simulink model "sharedControlBackup"  (R2018a)
settings: Solver=FixedStepAuto  StartTime=0.0  StopTime=200  FixedStep=.1  RelTol=1e-3
values from neighbouring files (symbols this model uses):
  a = -real(s1) + imag(s1)/tan(angle(s1+b) - theta)    [RLDesignJoystick.m]    (also in gainPlot.m = 10)
  a1 = b1/K    [RLDesignJoystick.m]
  b = 1.2*bb/I    (= 0.4)    [RLDesignJoystick.m]    (also in gainPlot.m)
  b1 = -real(s1)/150    [RLDesignJoystick.m]
  K0 = abs(s1+a)/abs(Gs1)/abs(s1+b)    [RLDesignJoystick.m]    (also in gainPlot.m = 0.5)
  K1 = 1/abs(Gs1)    [RLDesignJoystick.m]
undefined symbols (not defined in the file or in its folder): a2, b2, K2, U
libraries: robotlib x4, simulink x1
settings Model: Creator=transmogrifierlight  LastModifiedBy=transmogrifier

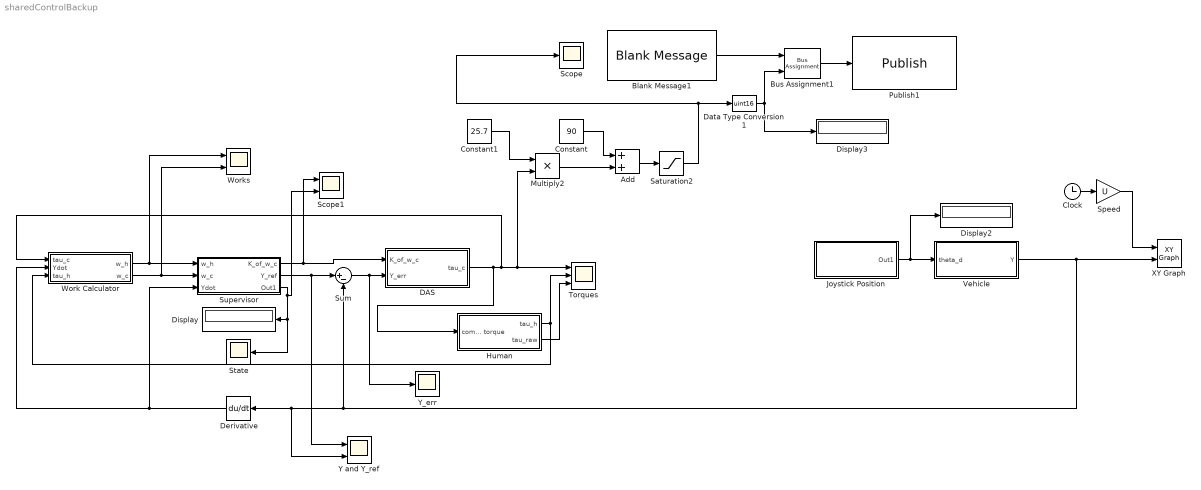
== system sharedControlBackup ==
  Add : Sum
  Blank Message1 : robotlib/Blank Message  SourceLibraryInfo=This block requires Robotics System Toolbox  messageType=std_msgs/UInt16  SampleTime=inf
      settings: SourceProductBaseCode=RO
  Bus Assignment1 : BusAssignment  AssignedSignals=Data
  Clock : Clock
  Constant : Constant  Value=90
  Constant1 : Constant  Value=25.7
  DAS : Subsystem
  Data Type Conversion1 : DataTypeConversion  OutDataTypeStr=uint16
  Derivative : Derivative
  Display : Display
  Display2 : Display
  Display3 : Display
  Human : Subsystem
  Joystick Position : Subsystem
  Multiply2 : Product
  Publish1 : robotlib/Publish  SourceLibraryInfo=This block requires Robotics System Toolbox  topicSource=Select from ROS network  topic=/yMotor  messageType=std_msgs/UInt16  messageQueueLength=1
      settings: SourceProductBaseCode=RO
  Saturation2 : Saturate  UpperLimit=140  LowerLimit=40
  Scope : Scope
  Scope1 : Scope  NumInputPorts=2
  Speed : Gain  Gain=U
  State : Scope
  Sum : Sum  Inputs=|+-
  Supervisor : Subsystem  mask{gamma_1_sq=0.2, gamma_2_sq=0.1, a_d=10, b_d=0.4, sigma_sq=0.1, delta_y=4, K3=0.5}
      mask prompts: gamma_1_sq "DAS Threshold"; gamma_2_sq "Human Threshold"; a_d "a"; b_d "b"; sigma_sq "Lane Change Threshold"; delta_y "Lane Change Delta"; K3 "K0"
  Torques : Scope  NumInputPorts=3
  Vehicle : Subsystem
  Work Calculator : Subsystem  mask{DT=4}
      mask prompts: DT "Time Window"
  Works : Scope  NumInputPorts=2
  XY Graph : simulink/Sinks/XY Graph  xmin=-10  xmax=U*200  ymin=-10  ymax=10  st=-1
  Y and Y_ref : Scope  NumInputPorts=2
  Y_err : Scope
  wires:
  Work Calculator/1(w_h) -> Works/1, Supervisor/1(w_h)
  Work Calculator/2(w_c) -> Works/2, Supervisor/2(w_c)
  Supervisor/1(K_of_w_c) -> Scope1/1, DAS/1("K_of_w_c ")
  Supervisor/2(Y_ref) -> Y and Y_ref/1, Sum/1
  Sum/1 -> Y_err/1, DAS/2(Y_err)
  Clock/1 -> Speed/1
  Speed/1 -> XY Graph/1
  Vehicle/1(Y) -> Sum/2, Y and Y_ref/2, Derivative/1, XY Graph/2
  Derivative/1 -> Work Calculator/2(Ydot), Supervisor/3(Ydot)
  Supervisor/3(Out1) -> Scope1/2, State/1, Display/1
  Human/1(tau_h) -> Work Calculator/3(tau_h), Torques/2
  Joystick Position/1(Out1) -> Vehicle/1(theta_d), Display2/1
  Bus Assignment1/1 -> Publish1/1
  Blank Message1/1 -> Bus Assignment1/1
  Data Type Conversion1/1 -> Bus Assignment1/2, Display3/1
  Constant1/1 -> Multiply2/1
  DAS/1(tau_c) -> Human/1(command torque), Work Calculator/1(tau_c), Multiply2/2, Torques/1
  Multiply2/1 -> Add/2
  Add/1 -> Saturation2/1
  Constant/1 -> Add/1
  Saturation2/1 -> Scope/1, Data Type Conversion1/1
  Human/2(tau_raw) -> Torques/3

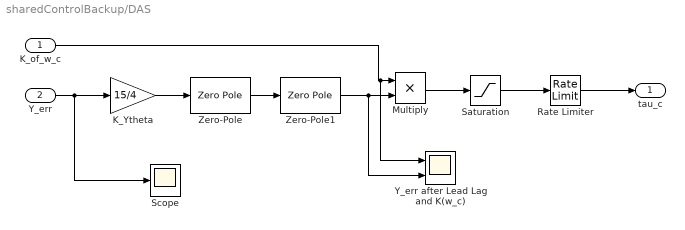
== system sharedControlBackup/DAS ==
  "K_of_w_c " : Inport
  Y_err : Inport  Port=2
  K_Ytheta : Gain  Gain=15/4
  Multiply : Product
  Rate Limiter : RateLimiter  RisingSlewLimit=3  FallingSlewLimit=-3  SampleTimeMode=inherited
  Saturation : Saturate  UpperLimit=5  LowerLimit=-5
  Scope : Scope
  Y_err after Lead Lag and K(w_c) : Scope  NumInputPorts=2
  Zero-Pole : ZeroPole  Zeros=[-b]  Poles=[-a]  Gain=[K0]
  Zero-Pole1 : ZeroPole  Zeros=[-b1]  Poles=[-a1]  Gain=[K1]
  tau_c : Outport
  wires:
  Y_err/1 -> Scope/1, K_Ytheta/1
  Saturation/1 -> Rate Limiter/1
  Multiply/1 -> Saturation/1
  "K_of_w_c "/1 -> Y_err after Lead Lag and K(w_c)/1, Multiply/1
  Zero-Pole/1 -> Zero-Pole1/1
  K_Ytheta/1 -> Zero-Pole/1
  Zero-Pole1/1 -> Y_err after Lead Lag and K(w_c)/2, Multiply/2
  Rate Limiter/1 -> tau_c/1

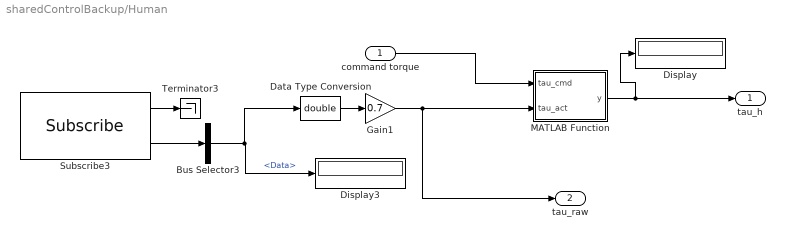
== system sharedControlBackup/Human ==
  command torque : Inport
  Bus Selector3 : BusSelector  OutputSignals=Data
  Data Type Conversion : DataTypeConversion  OutDataTypeStr=double
  Display : Display
  Display3 : Display
  Gain1 : Gain  Gain=0.7
  MATLAB Function : MATLAB Function  TreatAsAtomicUnit=on
  Subscribe3 : robotlib/Subscribe  SourceLibraryInfo=This block requires Robotics System Toolbox  topicSource=Select from ROS network  topic=/yCurrent  messageType=std_msgs/Float32  sampleTime=-1  messageQueueLength=1
      settings: SourceProductBaseCode=RO
  Terminator3 : Terminator
  tau_h : Outport
  tau_raw : Outport  Port=2
  wires:
  Subscribe3/1 -> Terminator3/1
  Data Type Conversion/1 -> Gain1/1
  Subscribe3/2 -> Bus Selector3/1
  Bus Selector3/1 -> Data Type Conversion/1, Display3/1  "<Data>"
  Gain1/1 -> tau_raw/1, MATLAB Function/2(tau_act)
  command torque/1 -> MATLAB Function/1(tau_cmd)
  MATLAB Function/1(y) -> Display/1, tau_h/1

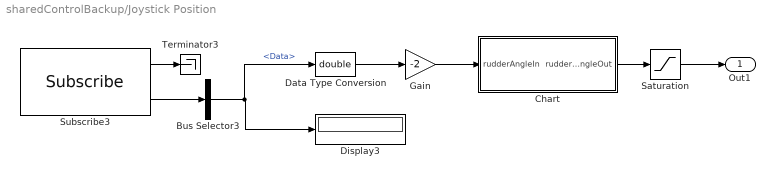
== system sharedControlBackup/Joystick Position ==
  Bus Selector3 : BusSelector  OutputSignals=Data
  Chart : Stateflow chart  TreatAsAtomicUnit=on
  Data Type Conversion : DataTypeConversion  OutDataTypeStr=double
  Display3 : Display
  Gain : Gain  Gain=-2
  Saturation : Saturate  UpperLimit=20  LowerLimit=-20
  Subscribe3 : robotlib/Subscribe  SourceLibraryInfo=This block requires Robotics System Toolbox  topicSource=Select from ROS network  topic=/yPos  messageType=std_msgs/Float32  sampleTime=-1  messageQueueLength=1
      settings: SourceProductBaseCode=RO
  Terminator3 : Terminator
  Out1 : Outport
  wires:
  Subscribe3/2 -> Bus Selector3/1
  Subscribe3/1 -> Terminator3/1
  Bus Selector3/1 -> Data Type Conversion/1, Display3/1  "<Data>"
  Data Type Conversion/1 -> Gain/1
  Gain/1 -> Chart/1(rudderAngleIn)
  Chart/1(rudderAngleOut) -> Saturation/1
  Saturation/1 -> Out1/1

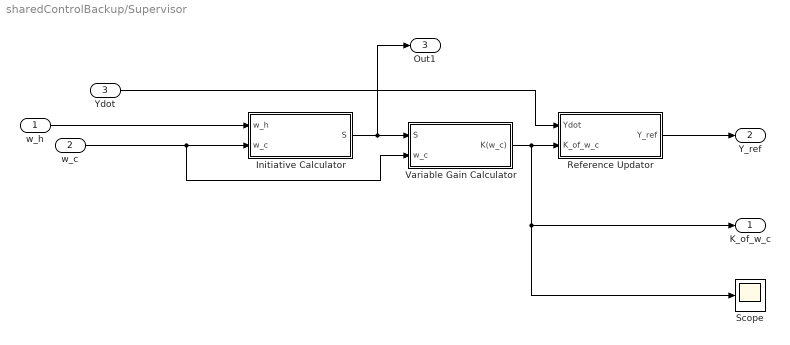
== system sharedControlBackup/Supervisor ==
  w_h : Inport
  w_c : Inport  Port=2
  Ydot : Inport  Port=3
  Initiative Calculator : Subsystem
  Reference Updator : Subsystem
  Scope : Scope
  Variable Gain Calculator : Subsystem
  K_of_w_c : Outport
  Y_ref : Outport  Port=2
  Out1 : Outport  Port=3
  wires:
  w_c/1 -> Variable Gain Calculator/2(w_c), Initiative Calculator/2("w_c ")
  w_h/1 -> Initiative Calculator/1(w_h)
  Initiative Calculator/1(S) -> Out1/1, Variable Gain Calculator/1(S)
  Variable Gain Calculator/1(K(w_c)) -> Reference Updator/2(K_of_w_c), Scope/1, K_of_w_c/1
  Ydot/1 -> Reference Updator/1(Ydot)
  Reference Updator/1(Y_ref) -> Y_ref/1

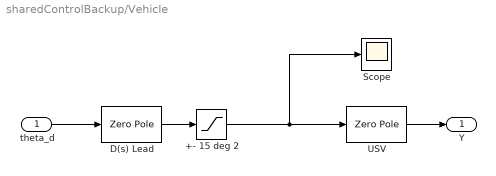
== system sharedControlBackup/Vehicle ==
  theta_d : Inport
  +- 15 deg 2 : Saturate  UpperLimit=20  LowerLimit=-20
  D(s) Lead : ZeroPole  Zeros=[-b2]  Poles=[-a2]  Gain=[K2]
  Scope : Scope
  USV : ZeroPole  Zeros=[]  Poles=[0 -5/4]  Gain=[1.5*1e-2]
  Y : Outport
  wires:
  USV/1 -> Y/1
  theta_d/1 -> D(s) Lead/1
  D(s) Lead/1 -> +- 15 deg 2/1
  +- 15 deg 2/1 -> USV/1, Scope/1

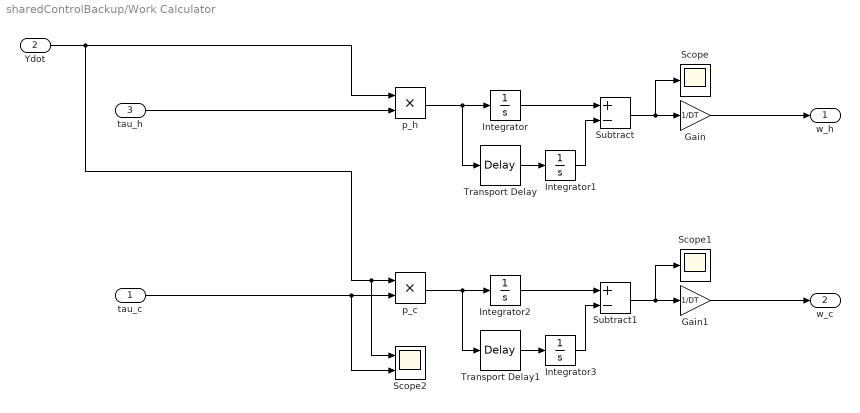
== system sharedControlBackup/Work Calculator ==
  tau_c : Inport
  Ydot : Inport  Port=2
  tau_h : Inport  Port=3
  Gain : Gain  Gain=1/DT
  Gain1 : Gain  Gain=1/DT
  Integrator{,1..3} (4 alike) : Integrator
  Scope : Scope
  Scope1 : Scope
  Scope2 : Scope  NumInputPorts=2
  Subtract : Sum  Inputs=+-
  Subtract1 : Sum  Inputs=+-
  Transport Delay : TransportDelay  DelayTime=DT
  Transport Delay1 : TransportDelay  DelayTime=DT
  p_c : Product
  p_h : Product
  w_h : Outport
  w_c : Outport  Port=2
  wires:
  tau_c/1 -> Scope2/2, p_c/2
  tau_h/1 -> p_h/2
  p_h/1 -> Transport Delay/1, Integrator/1
  Subtract/1 -> Scope/1, Gain/1
  Ydot/1 -> p_h/1, Scope2/1, p_c/1
  Transport Delay/1 -> Integrator1/1
  Integrator/1 -> Subtract/1
  Integrator1/1 -> Subtract/2
  Gain/1 -> w_h/1
  p_c/1 -> Transport Delay1/1, Integrator2/1
  Transport Delay1/1 -> Integrator3/1
  Subtract1/1 -> Scope1/1, Gain1/1
  Integrator2/1 -> Subtract1/1
  Integrator3/1 -> Subtract1/2
  Gain1/1 -> w_c/1

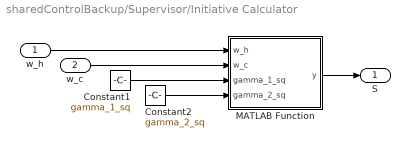
== system sharedControlBackup/Supervisor/Initiative Calculator ==
  w_h : Inport
  "w_c " : Inport  Port=2
  Constant1 : Constant  Value=gamma_1_sq
  Constant2 : Constant  Value=gamma_2_sq
  MATLAB Function : MATLAB Function  TreatAsAtomicUnit=on
  S : Outport
  wires:
  w_h/1 -> MATLAB Function/1(w_h)
  MATLAB Function/1(y) -> S/1
  Constant2/1 -> MATLAB Function/4(gamma_2_sq)
  "w_c "/1 -> MATLAB Function/2(w_c)
  Constant1/1 -> MATLAB Function/3(gamma_1_sq)

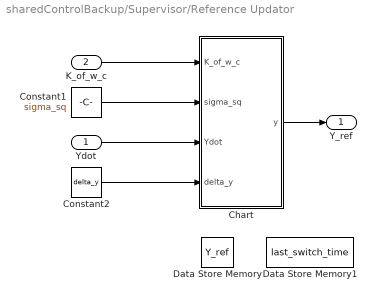
== system sharedControlBackup/Supervisor/Reference Updator ==
  Ydot : Inport
  K_of_w_c : Inport  Port=2
  Chart : Stateflow chart  TreatAsAtomicUnit=on
  Constant1 : Constant  Value=sigma_sq
  Constant2 : Constant  Value=delta_y
  Data Store Memory : DataStoreMemory  DataStoreName=Y_ref  ReadBeforeWriteMsg=warning  WriteAfterWriteMsg=warning  WriteAfterReadMsg=warning  ShowAdditionalParam=off  OutDataTypeStr=int16
  Data Store Memory1 : DataStoreMemory  DataStoreName=last_switch_time  ReadBeforeWriteMsg=warning  WriteAfterWriteMsg=warning  WriteAfterReadMsg=warning  ShowAdditionalParam=off  OutDataTypeStr=double
  Y_ref : Outport
  wires:
  Ydot/1 -> Chart/3(Ydot)
  K_of_w_c/1 -> Chart/1(K_of_w_c)
  Chart/1(y) -> Y_ref/1
  Constant1/1 -> Chart/2(sigma_sq)
  Constant2/1 -> Chart/4(delta_y)

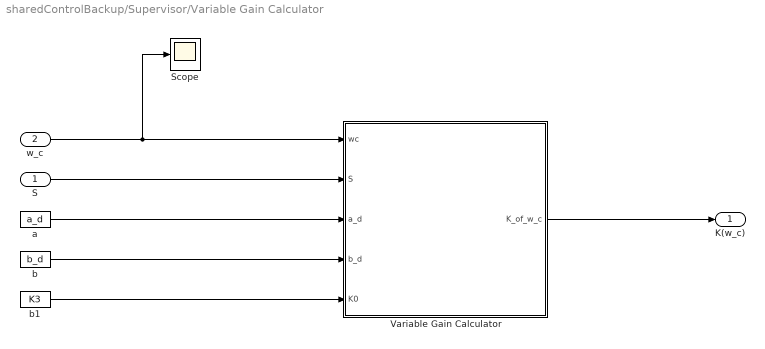
== system sharedControlBackup/Supervisor/Variable Gain Calculator ==
  S : Inport
  w_c : Inport  Port=2
  Scope : Scope
  "Variable Gain Calculator " : MATLAB Function  TreatAsAtomicUnit=on
  a : Constant  Value=a_d
  b : Constant  Value=b_d
  b1 : Constant  Value=K3
  K(w_c) : Outport
  wires:
  "Variable Gain Calculator "/1(K_of_w_c) -> K(w_c)/1
  a/1 -> "Variable Gain Calculator "/3(a_d)
  w_c/1 -> Scope/1, "Variable Gain Calculator "/1(wc)
  S/1 -> "Variable Gain Calculator "/2(S)
  b/1 -> "Variable Gain Calculator "/4(b_d)
  b1/1 -> "Variable Gain Calculator "/5(K0)

== stateflow chart sharedControlBackup/Supervisor/Reference Updator/Chart ==
  note: This system will check if there should be a lane changed
      | based on K(w_c) vs siqma^2.  If a lane change is required,
      | check to see if allowed based on time since last lane change
  note: C style logic:
      | if(K_of_w_c<=sigma_sq)
      | if(Ydot>0)
      | Y_ref=Y_ref+delta_y;
      | elseif(Ydot<0)
      | Y_ref=Y_ref-delta_y;
      | end
      | end
      | y = Y_ref;
  state add
    entry:Y_ref=Y_ref+delta_y;
    y=Y_ref;
    set_last_switch_time;
  state checkForChange
    entry: change_flag=time_check(5);
  state subtract
    entry:Y_ref=Y_ref-delta_y;
    y=Y_ref;
    set_last_switch_time;
  note: T_min=5
  add -> checkForChange
  (default) -> checkForChange
  (junction 47) -> add [order 1] : [Ydot>0]
  checkForChange -> (junction 44) [order 1] : [change_flag==true]
  (junction 44) -> (junction 47) [order 1] : [(K_of_w_c<=sigma_sq)]
  (junction 44) -> checkForChange [order 2] : [(K_of_w_c>sigma_sq)]
  (junction 47) -> subtract [order 2] : [Ydot<0]
  checkForChange -> checkForChange [order 2] : [change_flag==false]
  subtract -> checkForChange
  data: change function_output; t_min function_input; K_of_w_c input; sigma_sq input; y output; Ydot input; delta_y input; Y_ref data_store_memory; last_switch_time data_store_memory; current_time local; change_flag local
  function change=time_check(t_min):
    | function change=time_check(t_min)
    | global last_switch_time
    | coder.extrinsic('get_param');
    | temp=0;
    | temp=get_param('sharedControlWOControllers','SimulationTime');
    | change=(temp-last_switch_time)>t_min;
  function set_last_switch_time:
    | function set_last_switch_time
    | global last_switch_time
    | coder.extrinsic('get_param')
    | last_switch_time=get_param('sharedControlWOControllers','SimulationTime');

== matlab function sharedControlBackup/Supervisor/Initiative Calculator/MATLAB Function ==
  data: w_h input; y output; w_c input; gamma_1_sq input; gamma_2_sq input
function y = fcn(w_h, w_c, gamma_1_sq, gamma_2_sq)

if(w_h >= -gamma_1_sq && w_c >= -gamma_2_sq)
    S=1;
elseif(w_h >= -gamma_1_sq && w_c < -gamma_2_sq)
    S=2;
elseif(w_h < -gamma_1_sq && w_c >= -gamma_2_sq)
    S=3;
elseif(w_h < -gamma_1_sq && w_c < -gamma_2_sq)
    S=4;
else
    error('bad state assignment');
end
y = S;

== matlab function sharedControlBackup/Supervisor/Variable Gain Calculator/Variable Gain Calculator  ==
  data: wc input; S input; K_of_w_c output; a_d input; b_d input; K0 input
function K_of_w_c = fcn(wc, S, a_d, b_d, K0)

if S == 2    
    K_of_w_c = K0/(1 + exp(-a_d*wc + b_d));
else
    K_of_w_c = K0;
end

return

== stateflow chart sharedControlBackup/Joystick Position/Chart ==
  state zero_band
    entry:
    rudderAngleOut=0;
  state normal_operation
    entry:
    rudderAngleOut=rudderAngleIn;
  (default) -> zero_band
  zero_band -> normal_operation : [rudderAngleIn>=2||rudderAngleIn<=-2]
  normal_operation -> zero_band [order 1] : [rudderAngleIn<2&&rudderAngleIn>-2]
  normal_operation -> normal_operation [order 2]
  data: rudderAngleIn input; rudderAngleOut output

== matlab function sharedControlBackup/Human/MATLAB Function ==
  data: tau_cmd input; tau_act input; y output
function y = fcn(tau_cmd, tau_act)
if (tau_act>=0&&tau_act<4) || (tau_act<=0&&tau_act>-4)
    y=0;
else
    y=tau_act-tau_cmd;
end
